simulink model "tut2_2"  (R2018b)
settings: Solver=VariableStepAuto  StartTime=0.0  StopTime=60  RelTol=1e-3
values from neighbouring files (symbols this model uses):
  Kd = 5/4    (= 1.25)    [tut2.m]
  Ki = 9/6    (= 1.5)    [tut2.m]
  Kp = 7/4    (= 1.75)    [tut2.m]
  s = tf('s')    [tut2.m]
  tauD = 1/6    (= 0.166666666667)    [tut2.m]
libraries: cstblocks x6
settings Model: Creator=c3277928  LastModifiedBy=c3277928

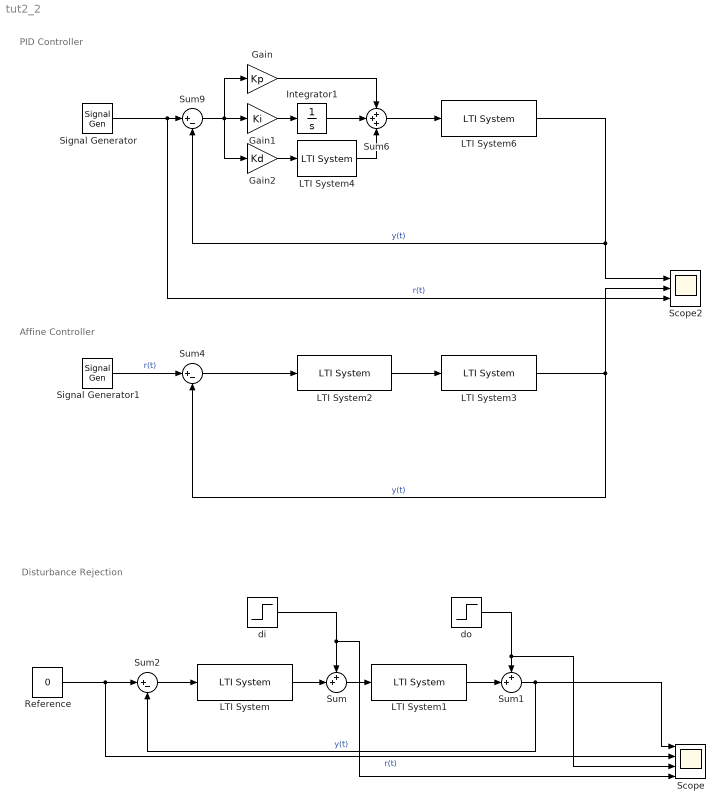
== system tut2_2 ==
  note: Affine Controller
  note: PID Controller
  note: Disturbance Rejection
  Gain : Gain  Gain=Kp
  Gain1 : Gain  Gain=Ki
  Gain2 : Gain  Gain=Kd
  Integrator1 : Integrator
  LTI System : cstblocks/LTI System  sys=C  IC=[]
  LTI System1 : cstblocks/LTI System  sys=G  IC=[]
  LTI System2 : cstblocks/LTI System  sys=C  IC=[]
  LTI System3 : cstblocks/LTI System  sys=G  IC=[]
  LTI System4 : cstblocks/LTI System  sys=s/(s+1/tauD)  IC=[]
  LTI System6 : cstblocks/LTI System  sys=G  IC=[]
  "Reference " : Constant  Value=0
  Scope : Scope  NumInputPorts=4
  Scope2 : Scope  NumInputPorts=3
  Signal Generator : SignalGenerator  WaveForm=square  Frequency=0.2
  Signal Generator1 : SignalGenerator  WaveForm=square  Frequency=0.2
  Sum : Sum  Inputs=++|
  Sum1 : Sum  Inputs=++|
  Sum2 : Sum  Inputs=|+-
  Sum4 : Sum  Inputs=|+-
  Sum6 : Sum  Inputs=+++
  Sum9 : Sum  Inputs=|+-
  "di " : Step  Time=20  SampleTime=0
  "do " : Step  Time=40  SampleTime=0
  wires:
  Sum/1 -> LTI System1/1
  LTI System/1 -> Sum/2
  LTI System1/1 -> Sum1/2
  Sum1/1 -> Sum2/2, Scope/1  "y(t)"
  Sum2/1 -> LTI System/1
  "di "/1 -> Scope/4, Sum/1
  "do "/1 -> Scope/3, Sum1/1
  "Reference "/1 -> Scope/2, Sum2/1  "r(t)"
  Signal Generator/1 -> Scope2/3, Sum9/1  "r(t)"
  Sum9/1 -> Gain2/1, Gain/1, Gain1/1
  LTI System6/1 -> Sum9/2, Scope2/1  "y(t)"
  Sum6/1 -> LTI System6/1
  Gain/1 -> Sum6/1
  LTI System4/1 -> Sum6/3
  Gain2/1 -> LTI System4/1
  Integrator1/1 -> Sum6/2
  Gain1/1 -> Integrator1/1
  Signal Generator1/1 -> Sum4/1  "r(t)"
  LTI System3/1 -> Scope2/2, Sum4/2  "y(t)"
  Sum4/1 -> LTI System2/1
  LTI System2/1 -> LTI System3/1
